simulink model "bmc_product2"  (R2021a)
settings: Solver=FixedStepAuto  StartTime=0.0  StopTime=inf  RelTol=1e-3  EnableMultiTasking=on
values from neighbouring files (symbols this model uses):
  HEARTBEAT_THRESH = 75    [bmc_product2_param.m]
  HUMIDITY = 54    [bmc_product2_param.m]
  HUMIDITY_THRESH = 55    [bmc_product2_param.m]
  PPG_THRESH = 520    [bmc_product2_param.m]
  SAMPLE_TIME = 0.01    [bmc_product2_param.m]
  TEMPERATURE = 27    [bmc_product2_param.m]
  TEMPERATURE_THRESH = 28    [bmc_product2_param.m]
libraries: arduinolib x14, simulink x11, dspstat3 x7, dspswit3 x6, dspxfrm3 x1, dspsigops x1
settings Model: SILPILModeSetting=veronly  EnablePacing=on  ExtModeTrigDuration=2  Creator=yuuri moriyama  LastModifiedBy=yuuri moriyama
settings OptimizationCC: EnhancedBackFolding=on  PassReuseOutputArgsAs=Individual arguments  ZeroExternalMemoryAtStartup=off  ZeroInternalMemoryAtStartup=off  MaxStackSize=64  OptimizeBlockOrder=speed  DifferentSizesBufferReuse=on  OptimizationCustomize=off  EfficientTunableParamExpr=on
settings DebuggingCC: ParameterTunabilityLossMsg=error
settings HardwareCC: ProdBitPerInt=16  ProdBitPerPointer=16  ProdBitPerSizeT=16  ProdBitPerPtrDiffT=16  ProdLargestAtomicFloat=None  ProdWordSize=8  ProdHWDeviceType=Atmel->AVR  UseEmbeddedCoderFeatures=off
settings SFSimCC: MATLABDynamicMemAlloc=off
settings RTWCC: SystemTargetFile=ert.tlc  HardwareBoard=Arduino Uno  TemplateMakefile=ert_default_tmf  Toolchain=Arduino AVR  BuildConfiguration=Faster Runs
settings CodeAppCC: ForceParamTrailComments=on  IgnoreCustomStorageClasses=off  OperatorAnnotations=on  SimulinkDataObjDesc=on  SFDataObjDesc=on  InsertBlockDesc=on
settings ERTTargetCC: SupportContinuousTime=on  SupportNonInlinedSFcns=on  SupportVariableSizeSignals=on  ExtModeStaticAllocSize=250

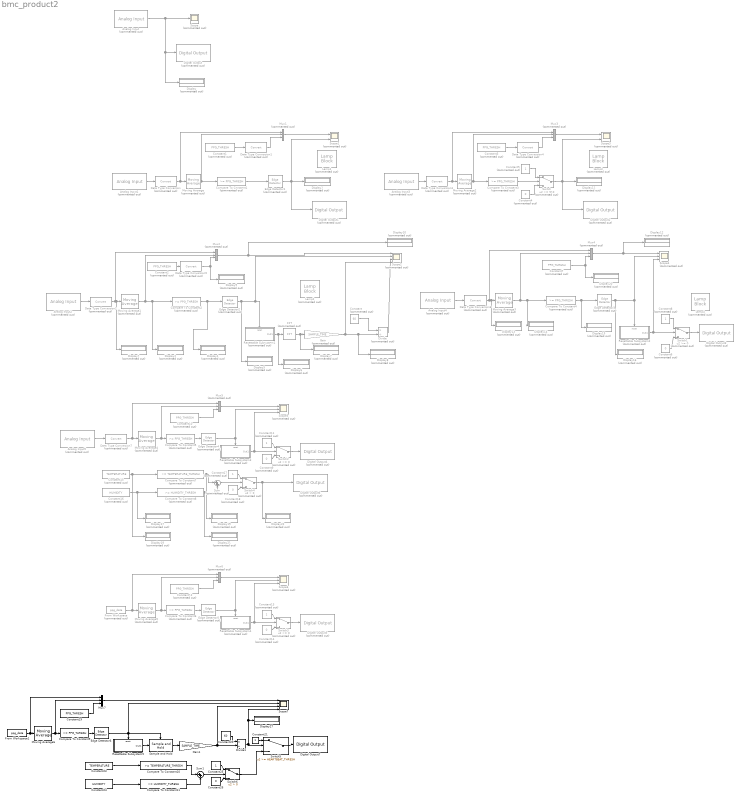
== system bmc_product2 ==
  Analog Input : arduinolib/Analog Input  Commented=on  pinNumber=4  ReadResultsOnly=off  ConversionTriggerSource=Software  ExternalTriggerType=uint32( 0 )  OutputDataType=uint16  EnableConversionCompleteNotify=off  EnableOuputStatus=off  SampleTime=-1  blockPlatform=arduino
  Analog Input{1..5} (5 alike) : arduinolib/Analog Input  Commented=on  pinNumber=0  ReadResultsOnly=off  ConversionTriggerSource=Software  ExternalTriggerType=uint32( 0 )  OutputDataType=uint16  EnableConversionCompleteNotify=off  EnableOuputStatus=off  SampleTime=-1  blockPlatform=arduino
  Compare To Constant1 : simulink/Logic and Bit Operations/Compare To Constant  Commented=on  relop=>=  const=PPG_THRESH  OutDataTypeStr=uint8
  Compare To Constant10 : simulink/Logic and Bit Operations/Compare To Constant  relop=>=  const=TEMPERATURE_THRESH  OutDataTypeStr=boolean
  Compare To Constant11 : simulink/Logic and Bit Operations/Compare To Constant  relop=>=  const=HUMIDITY_THRESH  OutDataTypeStr=boolean
  Compare To Constant{2,4..6} (4 alike) : simulink/Logic and Bit Operations/Compare To Constant  Commented=on  relop=>=  const=PPG_THRESH  OutDataTypeStr=boolean
  Compare To Constant3 : simulink/Logic and Bit Operations/Compare To Constant  Commented=on  relop=>=  const=PPG_THRESH  OutDataTypeStr=uint8
  Compare To Constant7 : simulink/Logic and Bit Operations/Compare To Constant  Commented=on  relop=>=  const=TEMPERATURE_THRESH  OutDataTypeStr=boolean
  Compare To Constant8 : simulink/Logic and Bit Operations/Compare To Constant  Commented=on  relop=>=  const=HUMIDITY_THRESH  OutDataTypeStr=boolean
  Compare To Constant9 : simulink/Logic and Bit Operations/Compare To Constant  relop=>=  const=PPG_THRESH  OutDataTypeStr=boolean
  Constant : Constant  Commented=on  Value=60
  Constant{1..3,7,10,12} (6 alike) : Constant  Commented=on  Value=PPG_THRESH
  Constant{5,8,11,13,17} (5 alike) : Constant  Commented=on
  Constant{4,6,9,14,18} (5 alike) : Constant  Commented=on  Value=0
  Constant15 : Constant  Commented=on  Value=TEMPERATURE
  Constant16 : Constant  Commented=on  Value=HUMIDITY
  Constant19 : Constant  Value=PPG_THRESH
  Constant20 : Constant  Value=60
  Constant21 : Constant
  Constant23 : Constant  Value=TEMPERATURE
  Constant24 : Constant  Value=HUMIDITY
  Constant25 : Constant
  Constant26 : Constant  Value=0
  Data Type Conversion{,1..7} (8 alike) : DataTypeConversion  Commented=on
  Digital Output{,1..6} (7 alike) : arduinolib/Digital Output  Commented=on  pinNumber=13  Direction=output  blockPlatform=arduino
  Digital Output7 : arduinolib/Digital Output  pinNumber=13  Direction=output  blockPlatform=arduino
  Display{,1..22} (23 alike) : Display  Commented=on
  Display27 : Display
  Divide : Product  Commented=on  Inputs=*/
  Divide1 : Product  Inputs=*/
  Edge Detector{1..5} (5 alike) : dspswit3/Edge Detector  Commented=on  InputProcessing=Columns as channels (frame based)
      settings: SourceProductBaseCode=DS
  Edge Detector6 : dspswit3/Edge Detector  InputProcessing=Columns as channels (frame based)
      settings: SourceProductBaseCode=DS
  FFT : dspxfrm3/FFT  Commented=on  FFTImplementation=Auto  CompMethod=Table lookup  TableOpt=NEW  TableOptActive=Speed  BitRevOrder=off  Normalize=off  InheritFFTLength=on  FFTLength=64  WrapInput=on  roundingMode=Floor  overflowMode=off  firstCoeffDataTypeStr=Inherit: Same word length as input  firstCoeffLastDataTypeStr=Inherit: Same word length as input  outputMin=[]  outputMax=[]
  From Workspace : FromWorkspace  Commented=on  VariableName=ppg_data  SampleTime=SAMPLE_TIME  Interpolate=off  OutputAfterFinalValue=Cyclic repetition
  From Workspace1 : FromWorkspace  VariableName=ppg_data  SampleTime=SAMPLE_TIME  Interpolate=off  OutputAfterFinalValue=Cyclic repetition
  Gain : Gain  Commented=on  Gain=SAMPLE_TIME
  Gain1 : Gain  Gain=SAMPLE_TIME
  Lamp{1..4} (4 alike) : LampBlock  Commented=on
  Moving Average{,1..5} (6 alike) : dspstat3/Moving Average  Commented=on  Method=Sliding window  ForgettingFactorPort=off  SpecifyWindowLength=on  WindowLength=4  ForgettingFactor=0.9  SimulateUsing=Code generation
  Moving Average6 : dspstat3/Moving Average  Method=Sliding window  ForgettingFactorPort=off  SpecifyWindowLength=on  WindowLength=4  ForgettingFactor=0.9  SimulateUsing=Code generation
  Mux{1..6} (6 alike) : Mux  Commented=on  Inputs=3
  Mux7 : Mux  Inputs=3
  Resettable Subsystem1 : Subsystem  Commented=on  TreatAsAtomicUnit=on
  Resettable Subsystem2 : Subsystem  Commented=on  TreatAsAtomicUnit=on
  Resettable Subsystem3 : Subsystem  Commented=on  TreatAsAtomicUnit=on
  Resettable Subsystem4 : Subsystem  Commented=on  TreatAsAtomicUnit=on
  Resettable Subsystem5 : Subsystem  TreatAsAtomicUnit=on
  Sample and Hold : dspsigops/Sample and Hold  trig=Rising edge  initCond=0  latchinput=on
  Scope : Scope  Commented=on
  Scope1 : Scope  Commented=on  NumInputPorts=2
  Scope2 : Scope  Commented=on  NumInputPorts=4
  Scope3 : Scope  Commented=on  NumInputPorts=2
  Scope4 : Scope  Commented=on  NumInputPorts=3
  Scope5 : Scope  Commented=on  NumInputPorts=3
  Scope6 : Scope  Commented=on  NumInputPorts=3
  Scope7 : Scope  NumInputPorts=4
  Sum : Sum  Commented=on  Inputs=|++
  Sum1 : Sum  Inputs=|++
  Switch : Switch  Commented=on  Threshold=510
  Switch1 : Switch  Commented=on
  Switch2 : Switch  Commented=on
  Switch3 : Switch  Commented=on
  Switch4 : Switch  Commented=on  Criteria=u2 > Threshold
  Switch5 : Switch  Threshold=HEARTBEAT_THRESH
  Switch6 : Switch  Criteria=u2 > Threshold
  wires:
  Analog Input/1 -> Display/1, Digital Output/1, Scope/1
  Data Type Conversion1/1 -> Mux1/3
  Data Type Conversion/1 -> Moving Average/1, Mux1/1
  Constant1/1 -> Data Type Conversion1/1
  Edge Detector1/1 -> Digital Output1/1, Scope1/2, Display1/1
  Mux1/1 -> Scope1/1
  Compare To Constant1/1 -> Edge Detector1/1
  Moving Average/1 -> Mux1/2, Compare To Constant1/1
  Analog Input1/1 -> Data Type Conversion/1
  Edge Detector2/1 -> Display5/1, Resettable Subsystem1/Reset, Scope2/2
  Resettable Subsystem1/1(Out1) -> FFT/1, Display6/1
  Mux2/1 -> Display10/1, Scope2/1
  Compare To Constant2/1 -> Display4/1, Edge Detector2/1
  FFT/1 -> Display7/1, Gain/1
  Moving Average1/1 -> Mux2/2, Display3/1, Compare To Constant2/1
  Gain/1 -> Scope2/4, Display8/1, Divide/2
  Constant/1 -> Divide/1
  Divide/1 -> Scope2/3
  Analog Input2/1 -> Data Type Conversion2/1
  Data Type Conversion2/1 -> Mux2/1, Display2/1, Moving Average1/1
  Moving Average2/1 -> Mux3/2, Compare To Constant3/1
  Mux3/1 -> Scope3/1
  Analog Input3/1 -> Data Type Conversion3/1
  Compare To Constant3/1 -> Switch/2
  Constant3/1 -> Data Type Conversion4/1
  Switch/1 -> Digital Output2/1, Scope3/2, Display11/1
  Data Type Conversion4/1 -> Mux3/3
  Data Type Conversion3/1 -> Moving Average2/1, Mux3/1
  Constant5/1 -> Switch/1
  Constant4/1 -> Switch/3
  Constant2/1 -> Data Type Conversion5/1
  Data Type Conversion5/1 -> Display9/1, Mux2/3
  Constant7/1 -> Display20/1, Mux4/3
  Analog Input4/1 -> Data Type Conversion6/1
  Data Type Conversion6/1 -> Mux4/1, Display13/1, Moving Average3/1
  Moving Average3/1 -> Mux4/2, Display14/1, Compare To Constant4/1
  Mux4/1 -> Display12/1, Scope4/1
  Edge Detector3/1 -> Display16/1, Resettable Subsystem2/Reset, Scope4/2
  Compare To Constant4/1 -> Display15/1, Edge Detector3/1
  Constant8/1 -> Switch1/1
  Resettable Subsystem2/1(Out1) -> Scope4/3, Switch1/2
  Constant6/1 -> Switch1/3
  Switch1/1 -> Digital Output3/1
  Constant11/1 -> Switch2/1
  Switch2/1 -> Digital Output4/1
  Resettable Subsystem3/1(Out1) -> Scope5/3, Switch2/2
  Edge Detector4/1 -> Resettable Subsystem3/Reset, Scope5/2
  Compare To Constant5/1 -> Edge Detector4/1
  Mux5/1 -> Scope5/1
  Moving Average4/1 -> Mux5/2, Compare To Constant5/1
  Constant9/1 -> Switch2/3
  Data Type Conversion7/1 -> Mux5/1, Moving Average4/1
  Analog Input5/1 -> Data Type Conversion7/1
  Constant10/1 -> Mux5/3
  Mux6/1 -> Scope6/1
  Compare To Constant6/1 -> Edge Detector5/1
  Switch3/1 -> Digital Output5/1
  Edge Detector5/1 -> Resettable Subsystem4/Reset, Scope6/2
  Constant13/1 -> Switch3/1
  Constant14/1 -> Switch3/3
  Resettable Subsystem4/1(Out1) -> Scope6/3, Switch3/2
  Constant12/1 -> Mux6/3
  From Workspace/1 -> Mux6/1, Moving Average5/1
  Moving Average5/1 -> Mux6/2, Compare To Constant6/1
  Constant15/1 -> Display18/1, Compare To Constant7/1
  Constant16/1 -> Display17/1, Compare To Constant8/1
  Sum/1 -> Switch4/2
  Constant18/1 -> Switch4/3
  Constant17/1 -> Switch4/1
  Switch4/1 -> Display22/1, Digital Output6/1
  Compare To Constant8/1 -> Display21/1, Sum/2
  Compare To Constant7/1 -> Display19/1, Sum/1
  Constant19/1 -> Mux7/3
  Moving Average6/1 -> Mux7/2, Compare To Constant9/1
  Compare To Constant9/1 -> Edge Detector6/1
  From Workspace1/1 -> Mux7/1, Moving Average6/1
  Mux7/1 -> Scope7/1
  Edge Detector6/1 -> Sample and Hold/Trigger, Scope7/2, Resettable Subsystem5/Reset
  Resettable Subsystem5/1(Out1) -> Sample and Hold/1
  Sample and Hold/1 -> Gain1/1
  Gain1/1 -> Scope7/3, Divide1/2
  Constant20/1 -> Divide1/1
  Divide1/1 -> Scope7/4, Display27/1, Switch5/2
  Switch6/1 -> Switch5/3
  Constant21/1 -> Switch5/1
  Switch5/1 -> Digital Output7/1
  Compare To Constant10/1 -> Sum1/1
  Sum1/1 -> Switch6/2
  Constant23/1 -> Compare To Constant10/1
  Constant24/1 -> Compare To Constant11/1
  Compare To Constant11/1 -> Sum1/2
  Constant26/1 -> Switch6/3
  Constant25/1 -> Switch6/1

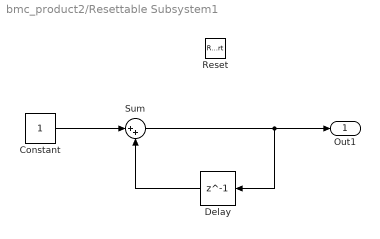
== system bmc_product2/Resettable Subsystem1 ==
  Reset : ResetPort  DisableCoverage=on
  Constant : Constant
  Delay : Delay  DelayLength=1  InitialCondition=0
  Sum : Sum  Inputs=|++
  Out1 : Outport
  wires:
  Constant/1 -> Sum/1
  Sum/1 -> Delay/1, Out1/1
  Delay/1 -> Sum/2

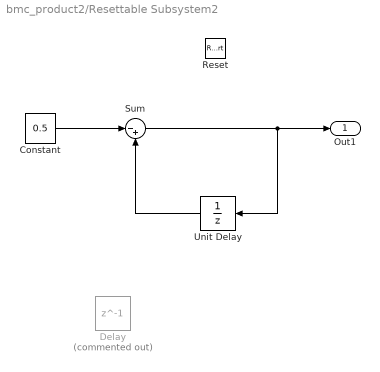
== system bmc_product2/Resettable Subsystem2 ==
  Reset : ResetPort  DisableCoverage=on
  Constant : Constant  Value=0.5
  Delay : Delay  Commented=on  DelayLength=1  InitialCondition=0
  Sum : Sum  Inputs=|-+
  Unit Delay : UnitDelay  InitialCondition=5  SampleTime=-1  HasFrameUpgradeWarning=on
  Out1 : Outport
  wires:
  Constant/1 -> Sum/1
  Sum/1 -> Unit Delay/1, Out1/1
  Unit Delay/1 -> Sum/2

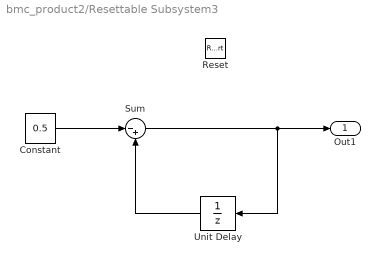
== system bmc_product2/Resettable Subsystem3 ==
  Reset : ResetPort  DisableCoverage=on
  Constant : Constant  Value=0.5
  Sum : Sum  Inputs=|-+
  Unit Delay : UnitDelay  InitialCondition=5  SampleTime=-1  HasFrameUpgradeWarning=on
  Out1 : Outport
  wires:
  Constant/1 -> Sum/1
  Sum/1 -> Unit Delay/1, Out1/1
  Unit Delay/1 -> Sum/2

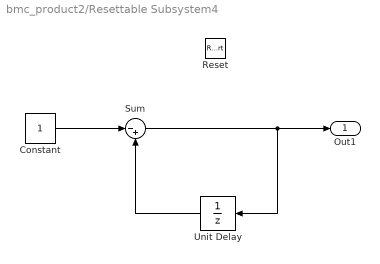
== system bmc_product2/Resettable Subsystem4 ==
  Reset : ResetPort  DisableCoverage=on
  Constant : Constant
  Sum : Sum  Inputs=|-+
  Unit Delay : UnitDelay  InitialCondition=80  SampleTime=-1  HasFrameUpgradeWarning=on
  Out1 : Outport
  wires:
  Constant/1 -> Sum/1
  Sum/1 -> Unit Delay/1, Out1/1
  Unit Delay/1 -> Sum/2

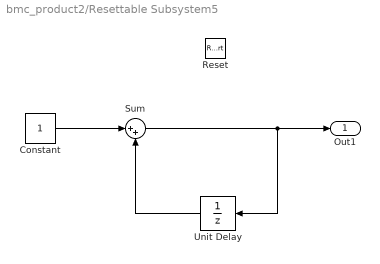
== system bmc_product2/Resettable Subsystem5 ==
  Reset : ResetPort  DisableCoverage=on
  Constant : Constant
  Sum : Sum  Inputs=|++
  Unit Delay : UnitDelay  SampleTime=-1  HasFrameUpgradeWarning=on
  Out1 : Outport
  wires:
  Constant/1 -> Sum/1
  Sum/1 -> Unit Delay/1, Out1/1
  Unit Delay/1 -> Sum/2
